simulink library "Vehicle_1Axle"  (R2019a)
settings: Solver=VariableStepAuto  StartTime=0.0  StopTime=10.0  RelTol=1e-3
undefined symbols (not defined in the file): Init, Trailer
libraries: sm_car_lib x5, sm_lib x1, $bdroot x1, Chassis_1Axle x1
Description:
  | Copyright 2020 The MathWorks, Inc.
settings Model: Creator=smiller  LastModifiedBy=smiller
settings DataIOCC: ReturnWorkspaceOutputs=off
settings DebuggingCC: ArithmeticOperatorsInVariantConditions=warning

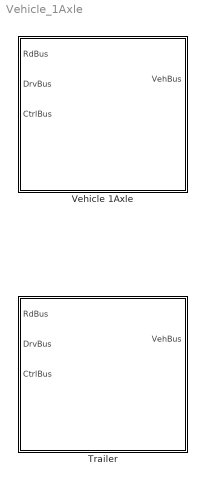
== system Vehicle_1Axle ==
  Trailer : Subsystem  VariantControlMode=Label  Variant=on  VariantControl=NS_Con  LabelModeActiveChoice=Trailer  mask{InitTriggerDropdown=0}
      mask prompts: InitTriggerDropdown "Mask Initialization Trigger"
      mask init:
      | curblk = gcb;
      | 
      | % Trigger Mask Initialization for 
      | % variant subsystems below this level
      | sm_car_lib_maskInitTrigger(curblk);
      mask TypeOptions InitTriggerDropdown: 0 | 1
      mask Display:
      | if(strcmpi(get_param(gcb,'LabelModeActiveChoice'),'Trailer'))
      |     trlvar = get_param([gcb '/Trailer'],'Vehicle');
      |     trlconfigstr = lower(evalin('base',[trlvar '.config']));
      |     trlstrings = strsplit(trlconfigstr,'_');
      |     temp_trailer_type = lower(trlstrings{1});
      |     if(strcmpi(temp_trailer_type,'thwala'))
      |         image(['sm_car_vehicle_trailer_' temp_trailer_type '_IMAGE.png']);
      |     else
      |         image('sm_car_vehicle_trailer_elula_IMAGE.png');
      |     end
      | end
  Vehicle 1Axle : Subsystem  Tag=PublishSubsystem  VariantControl=NS_Con  mask(Car){Vehicle=Trailer, Init=Init, InitTriggerDropdown=1}
      mask prompts: Vehicle "Vehicle Parameters"; Init "Initial Values"; InitTriggerDropdown "Initialization Trigger Dropdown"
      mask help: Vehicle model with multibody suspension. Change value of Initialization Trigger Dropdown to trigger selection of variant subsystems.
      mask init:
      | curblk = gcb;
      | 
      | % Trigger Mask Initialization for 
      | % variant subsystems below this level
      | sm_car_lib_maskInitTrigger(curblk)
      mask Help: web('sm_car_doc_vehicle.html')
      mask TypeOptions InitTriggerDropdown: 0 | 1
      mask DialogControl cont_sim Prompt: Config
      mask Display:
      | veh_param = get_param(gcb,'Vehicle');
      | veh_config = evalin('base',[veh_param '.config']);
      | veh_config_set = strsplit(veh_config,'_');
      | veh_body =  lower(veh_config_set{1});
      | 
      | if(strcmpi(veh_body,'thwala'))
      |     image(['sm_car_vehicle_trailer_' veh_body '_IMAGE.png']);
      | else
      |     image('sm_car_vehicle_trailer_elula_IMAGE.png');
      | end
      | 
      | %image('sm_car_vehicle_trailer_IMAGE.png');

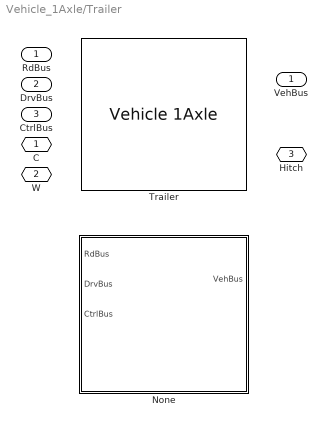
== system Vehicle_1Axle/Trailer ==
  "RdBus " : Inport
  "DrvBus " : Inport  Port=2
  "CtrlBus " : Inport  Port=3
  None : Subsystem  VariantControl=None
  Trailer : $bdroot/Vehicle 1Axle  Tag=PublishSubsystem  VariantControl=Trailer  Vehicle=Trailer  Init=Init_Trailer  InitTriggerDropdown=0
  " C" : PMIOPort  Side=Left
  " W" : PMIOPort  Port=2  Side=Left
  " Hitch" : PMIOPort  Port=3  Side=Right
  " VehBus" : Outport

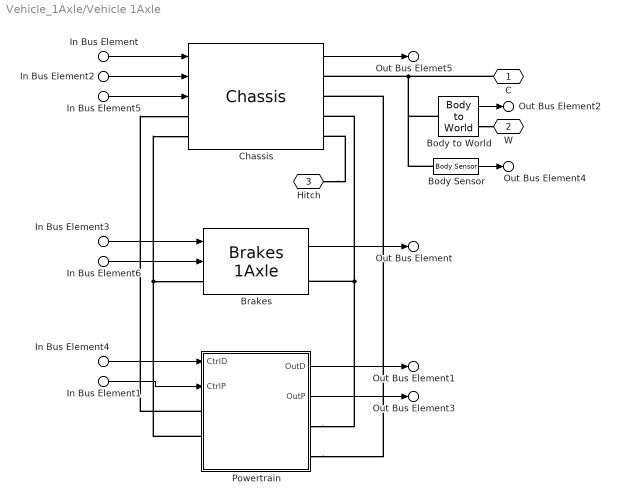
== system Vehicle_1Axle/Vehicle 1Axle ==
  In Bus Element2 : Inport  PortName=RdBus
  In Bus Element : Inport  Port=2  PortName=DrvBus
  In Bus Element3 : Inport  Port=2  PortName=DrvBus
  In Bus Element6 : Inport  Port=3  PortName=CtrlBus  Element=Brakes
  In Bus Element5 : Inport  Port=3  PortName=CtrlBus  Element=Chassis
  In Bus Element1 : Inport  Port=3  PortName=CtrlBus  Element=Power
  In Bus Element4 : Inport  Port=3  PortName=CtrlBus  Element=Driveline
  Body Sensor : sm_car_lib/Sensors/Body Sensor  SystemSampleTime=-1
  Body to World : sm_car_lib/Body/Body to World  Init=Init.Chassis  SpecifyPosTarget=off
  Brakes : sm_car_lib/Brakes/Brakes 1Axle  VariantControl=Variant1  Brakes=Vehicle.Brakes  VariantLabel=Vehicle.Brakes.class.Value  InitTriggerDropdown=1
      settings: AttributesFormatString=%<ActiveVariant>
  Chassis : Chassis_1Axle/Chassis  Tag=PublishSubsystem  VariantControl=Chassis  Chassis=Vehicle.Chassis  Init=Init  InitTriggerDropdown=1
  Powertrain : Subsystem  mask{Powertrain=Vehicle.Powertrain, InitTriggerDropdown=1}
      mask prompts: Powertrain "Powertrain Parameters"; InitTriggerDropdown "Initialization Trigger Dropdown"
      mask init:
      | curblk = gcb;
      | 
      | % Trigger Mask Initialization for 
      | % variant subsystems below this level
      | sm_car_lib_maskInitTrigger(curblk)
      mask TypeOptions InitTriggerDropdown: 0 | 1
  C : PMIOPort  Side=Left
  W : PMIOPort  Port=2  Side=Left
  Hitch : PMIOPort  Port=3  Side=Right
  Out Bus Element4 : Outport  PortName=VehBus  Element=Body
  Out Bus Elemet5 : Outport  PortName=VehBus  Element=Chassis
  Out Bus Element : Outport  PortName=VehBus  Element=Brakes
  Out Bus Element1 : Outport  PortName=VehBus  Element=Driveline
  Out Bus Element2 : Outport  PortName=VehBus  Element=World
  Out Bus Element3 : Outport  PortName=VehBus  Element=Power
  wires:
  Powertrain/2(OutP) -> Out Bus Element3/1
  Powertrain/1(OutD) -> Out Bus Element1/1
  In Bus Element1/1 -> Powertrain/2(CtrlP)
  In Bus Element4/1 -> Powertrain/1(CtrlD)
  In Bus Element3/1 -> Brakes/1
  Body to World/1 -> Out Bus Element2/1
  Body Sensor/1 -> Out Bus Element4/1
  In Bus Element6/1 -> Brakes/2
  In Bus Element/1 -> Chassis/1
  In Bus Element2/1 -> Chassis/2
  Chassis/1 -> Out Bus Elemet5/1
  Brakes/1 -> Out Bus Element/1
  In Bus Element5/1 -> Chassis/3
  connections:
  Powertrain/LConn1 -- Chassis/LConn1
  Powertrain/RConn2 -- Chassis/RConn2
  Powertrain/LConn2 -- Chassis/LConn2 -- Brakes/LConn1
  Powertrain/RConn1 -- Chassis/RConn3 -- Brakes/RConn1
  Body to World/RConn1 -- W/RConn1
  Body Sensor/LConn1 -- Body to World/LConn1 -- Chassis/RConn1 -- C/RConn1
  Hitch/RConn1 -- Chassis/RConn4

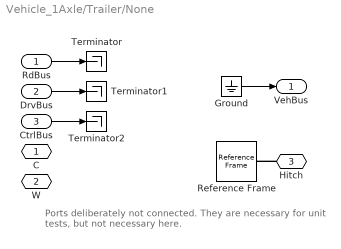
== system Vehicle_1Axle/Trailer/None ==
  note: Ports deliberately not connected. They are necessary for unit tests, but not necessary here.
  "RdBus " : Inport
  "DrvBus " : Inport  Port=2
  "CtrlBus " : Inport  Port=3
  Ground : Ground
  Reference Frame : sm_lib/Frames and Transforms/Reference Frame
  Terminator : Terminator
  Terminator1 : Terminator
  Terminator2 : Terminator
  " C" : PMIOPort  Side=Left
  " W" : PMIOPort  Port=2  Side=Left
  " Hitch" : PMIOPort  Port=3  Side=Right
  " VehBus" : Outport
  wires:
  "RdBus "/1 -> Terminator/1
  "DrvBus "/1 -> Terminator1/1
  "CtrlBus "/1 -> Terminator2/1
  Ground/1 -> " VehBus"/1
  connections:
  " Hitch"/RConn1 -- Reference Frame/RConn1

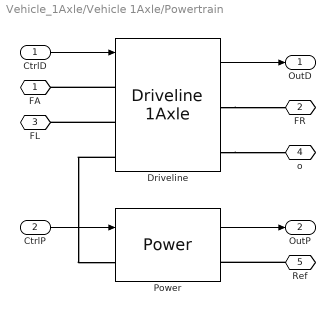
== system Vehicle_1Axle/Vehicle 1Axle/Powertrain ==
  CtrlD : Inport
  CtrlP : Inport  Port=2
  Driveline : sm_car_lib/Driveline/Driveline 1Axle  VariantControl=Shaft  Driveline=Vehicle.Powertrain.Driveline  VariantLabel=Vehicle.Powertrain.Driveline.class.Value  InitTriggerDropdown=1
      settings: AttributesFormatString=%<ActiveVariant>
  Power : sm_car_lib/Power/Power  VariantControl=Variant1  Power=Powertrain.Power  VariantLabel=Powertrain.Power.class.Value  InitTriggerDropdown=1
      settings: AttributesFormatString=%<ActiveVariant>
  FA : PMIOPort  Side=Left
  FR : PMIOPort  Port=2  Side=Right
  FL : PMIOPort  Port=3  Side=Left
  o : PMIOPort  Port=4  Side=Left
  Ref : PMIOPort  Port=5  Side=Right
  OutD : Outport
  OutP : Outport  Port=2
  wires:
  CtrlP/1 -> Power/1
  Power/1 -> OutP/1
  CtrlD/1 -> Driveline/1
  Driveline/1 -> OutD/1
  connections:
  Driveline/RConn2 -- o/RConn1
  Driveline/RConn1 -- FR/RConn1
  Driveline/LConn2 -- FL/RConn1
  Driveline/LConn3 -- Power/LConn1
  Ref/RConn1 -- Power/RConn1
  Driveline/LConn1 -- FA/RConn1
